simulink model "simulink_2018b"  (R2021a)
settings: Solver=ode4  StartTime=0.0  StopTime=t_f_window  FixedStep=0.0001  MaxStep=0.00002  MinStep=0.00001  RelTol=1e-7
values from neighbouring files (symbols this model uses):
  b_simulink = double(b)    [main.m]
  c_nom = double(c_nom)    [main.m]
  lambda_0_simulink = double(lambda_t_i_window)    [main.m]
  q_simulink = double(q)    [main.m]
  r_simulink = double(r)    [main.m]
  t_indices_simulink = double(t_indices_window)    [main.m]
  t_instants_simulink = double(t_window)    [main.m]
  u_nom = double(u_nom)    [main.m]
  w_pv_mean_simulink = double(w_pv_mean_window2)    [main.m]
  w_pv_real_simulink = double(w_pv(i:window+i))    [main.m]
  w_pv_simulink = double(w_pv_mean_window)    [main.m]
  w_r_mean_simulink = double(w_r_mean_window2)    [main.m]
  w_r_real_simulink = double(w_r(i:window+i))    [main.m]
  w_r_simulink = double(w_r_mean_window)    [main.m]
  w_r_variance_simulink = double(w_r_variance_window)    [main.m]
  x_t_i_simulink = double(x_t_i_window)    [main.m]
settings Model: Creator=Francesco  LastModifiedBy=emanuele
settings SolverCC: InitialStep=0.00001  AlgebraicLoopSolver=TrustRegion
settings DataIOCC: ReturnWorkspaceOutputs=off
settings DebuggingCC: SFMachineParentedDataDiag=warning  ArithmeticOperatorsInVariantConditions=warning
settings SFSimCC: CustomCodeUndefinedFunction=UseInterfaceOnly

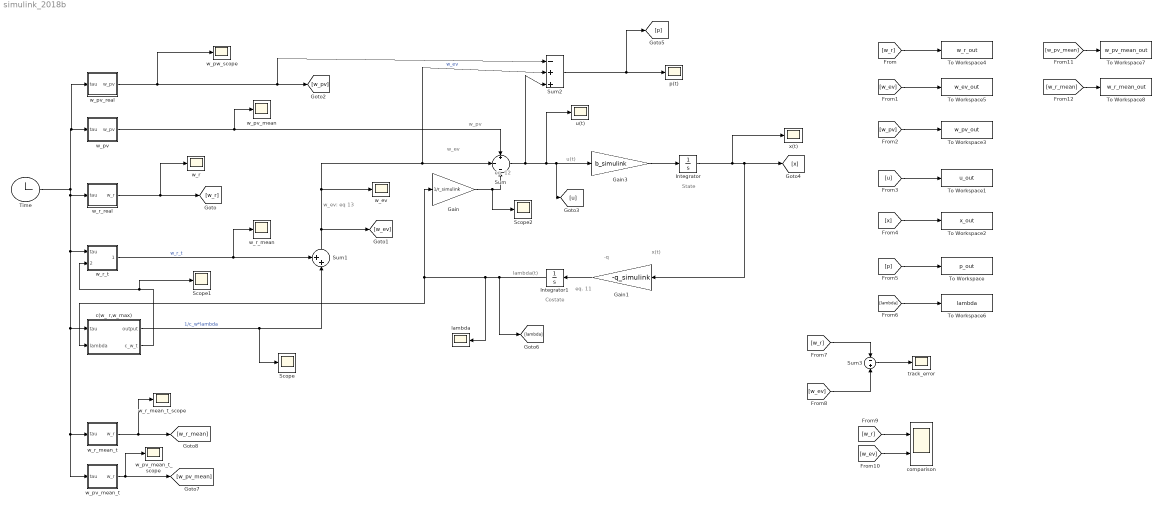
== system simulink_2018b ==
  note: w_ev:
      | eq 13
  note: eq. 11
  note: eq. 12
  note: Costate
  note: w_pv
  note: x(t)
  note: w_ev
  note: lambda(t)
  note: u(t)
  note: -q
  note: State
  Gain : Gain  Gain=1/r_simulink
  Gain1 : Gain  Gain=-q_simulink
  Gain3 : Gain  Gain=b_simulink
  Integrator : Integrator  InitialCondition=x_t_i_simulink
  Integrator1 : Integrator  InitialCondition=lambda_0_simulink
  Scope : Scope
  Scope1 : Scope
  Scope2 : Scope
  Sum : Sum  Inputs=+|-|-
  Sum1 : Sum  Inputs=++|
  Sum2 : Sum  Inputs=-++|
  Sum3 : Sum  Inputs=-+
  Time : Clock
  To Workspace : ToWorkspace  VariableName=p_out  SaveFormat=Timeseries  SampleTime=-1
  To Workspace1 : ToWorkspace  VariableName=u_out  SaveFormat=Timeseries  SampleTime=-1
  To Workspace2 : ToWorkspace  VariableName=x_out  SaveFormat=Timeseries  SampleTime=-1
  To Workspace3 : ToWorkspace  VariableName=w_pv_out  SaveFormat=Timeseries  SampleTime=-1
  To Workspace4 : ToWorkspace  VariableName=w_r_out  SaveFormat=Timeseries  SampleTime=-1
  To Workspace5 : ToWorkspace  VariableName=w_ev_out  SaveFormat=Timeseries  SampleTime=-1
  To Workspace6 : ToWorkspace  VariableName=lambda  SaveFormat=Timeseries  SampleTime=-1
  To Workspace7 : ToWorkspace  VariableName=w_pv_mean_out  SaveFormat=Timeseries  SampleTime=-1
  To Workspace8 : ToWorkspace  VariableName=w_r_mean_out  SaveFormat=Timeseries  SampleTime=-1
  c(w_ r,w_max) : MATLAB Function  TreatAsAtomicUnit=on
  comparison : Scope  NumInputPorts=2
  lambda : Scope
  p(t) : Scope
  track_error : Scope
  "u(t) " : Scope
  "w_ev " : Scope
  w_pv : MATLAB Function  TreatAsAtomicUnit=on
  w_pv_mean : Scope
  w_pv_mean_t : MATLAB Function  TreatAsAtomicUnit=on
  w_pv_mean_t_scope : Scope
  w_pv_real : MATLAB Function  TreatAsAtomicUnit=on
  w_pw_scope : Scope
  "w_r " : Scope
  w_r_mean : Scope
  w_r_mean_t : MATLAB Function  TreatAsAtomicUnit=on
  w_r_mean_t_scope : Scope
  w_r_real : MATLAB Function  TreatAsAtomicUnit=on
  w_r_t : MATLAB Function  TreatAsAtomicUnit=on
  "x(t) " : Scope
  wires:
  Gain/1 -> Scope2/1, Sum/3
  Integrator/1 -> "x(t) "/1, [x], Gain1/1
  Gain1/1 -> Integrator1/1
  Integrator1/1 -> [lambda], lambda/1, c(w_ r,w_max)/2(lambda), Gain/1
  Time/1 -> w_pv_mean_t/1(tau), w_r_mean_t/1(tau), c(w_ r,w_max)/1(tau), w_r_t/1(tau), w_r_real/1(tau), w_pv_real/1(tau), w_pv/1(tau)
  Gain3/1 -> Integrator/1
  Sum/1 -> Sum2/3, "u(t) "/1, [u], Gain3/1
  c(w_ r,w_max)/1(output) -> Scope/1, Sum1/2  "1/c_w*lambda"
  w_r_t/1(w_r_t) -> w_r_mean/1, Sum1/1  "w_r_t"
  Sum1/1 -> [w_ev], Sum2/2, Sum/2, "w_ev "/1  "w_ev"
  [w_r] -> To Workspace4/1
  [w_ev] -> To Workspace5/1
  [w_pv] -> To Workspace3/1
  [u] -> To Workspace1/1
  [x] -> To Workspace2/1
  [p] -> To Workspace/1
  Sum2/1 -> [p], p(t)/1
  w_pv/1(w_pv) -> Sum/1, w_pv_mean/1
  [lambda] -> To Workspace6/1
  Sum3/1 -> track_error/1
  [w_r] -> Sum3/1
  [w_ev] -> Sum3/2
  [w_r] -> comparison/1
  [w_ev] -> comparison/2
  c(w_ r,w_max)/2(c_w_t) -> Scope1/1, w_r_t/2(c_w_t)
  w_r_real/1(w_r) -> "w_r "/1, [w_r]
  w_pv_real/1(w_pv) -> Sum2/1, [w_pv], w_pw_scope/1
  [w_pv_mean] -> To Workspace7/1
  [w_r_mean] -> To Workspace8/1
  w_r_mean_t/1(w_r) -> w_r_mean_t_scope/1, [w_r_mean]
  w_pv_mean_t/1(w_r) -> w_pv_mean_t_scope/1, [w_pv_mean]

== matlab function simulink_2018b/w_r_t ==
  data: tau input; c_w_t input; w_r_simulink parameter; t_instants_simulink parameter; w_r_t output; t_indices_simulink parameter; c_nom parameter; u_nom parameter; w_r_variance_simulink parameter
function w_r_t = fcn(tau, c_w_t, w_r_simulink, t_instants_simulink, t_indices_simulink, c_nom, u_nom, w_r_variance_simulink)
    app=1;
    for i = 1:t_indices_simulink(end)-1
        if ( t_instants_simulink(i)<=tau )&&( tau<t_instants_simulink(i+1) )
            app = i;
            %break;
        end
    end
    E_w_r_square = w_r_simulink(app)^2 + w_r_variance_simulink(app);
    w_r_t = -(1/c_w_t)*c_nom*(E_w_r_square - (1+u_nom)*w_r_simulink(app));
    %w_r_t = w_r_simulink(app);
end

== matlab function simulink_2018b/w_pv ==
  data: tau input; w_pv output; w_pv_simulink parameter; t_instants_simulink parameter; t_indices_simulink parameter

%% profilo fotovoltaico - nullo per ora per semplicità
function w_pv = fcn(tau, w_pv_simulink, t_instants_simulink, t_indices_simulink)
    app=1;
    for i = 1:t_indices_simulink(end)-1
        if ( t_instants_simulink(i)<=tau )&&( tau<t_instants_simulink(i+1) )
            app = i;
            %break;
        end
    end
    w_pv = w_pv_simulink(app);
end

== matlab function simulink_2018b/c(w_ r,w_max) ==
  data: tau input; output output; lambda input; w_r_simulink parameter; t_indices_simulink parameter; t_instants_simulink parameter; c_w_t output; c_nom parameter; u_nom parameter
function [output, c_w_t] = fcn(tau, lambda, w_r_simulink, t_indices_simulink, t_instants_simulink, c_nom, u_nom)    
    app = 1;
    for i = 1:t_indices_simulink(end)-1
        if ( t_instants_simulink(i)<=tau )&&( tau<t_instants_simulink(i+1) )
            app = i;
        end
    end
    %c_w = assign_cw(w_r_simulink(app), p_cw_base_simulink, cw_base_simulink);
    c_w = c_nom * (1 + u_nom - w_r_simulink(app));
    output = (1/c_w)*lambda;
    c_w_t = c_w;
end
%% vedere se coeff_1 va riportato qui

== matlab function simulink_2018b/w_r_real ==
  data: tau input; w_r output; w_r_real_simulink parameter; t_instants_simulink parameter; t_indices_simulink parameter

%% profilo fotovoltaico - nullo per ora per semplicità
function w_r = fcn(tau, w_r_real_simulink, t_instants_simulink, t_indices_simulink)
    app=1;
    for i = 1:t_indices_simulink(end)-1
        if ( t_instants_simulink(i)<=tau )&&( tau<t_instants_simulink(i+1) )
            app = i;
            %break;
        end
    end
    w_r = w_r_real_simulink(app);
end

== matlab function simulink_2018b/w_pv_real ==
  data: tau input; w_pv output; w_pv_real_simulink parameter; t_instants_simulink parameter; t_indices_simulink parameter

%% profilo fotovoltaico - nullo per ora per semplicità
function w_pv = fcn(tau, w_pv_real_simulink, t_instants_simulink, t_indices_simulink)
    app=1;
    for i = 1:t_indices_simulink(end)-1
        if ( t_instants_simulink(i)<=tau )&&( tau<t_instants_simulink(i+1) )
            app = i;
            %break;
        end
    end
    w_pv = w_pv_real_simulink(app);
end

== matlab function simulink_2018b/w_r_mean_t ==
  data: tau input; w_r output; w_r_mean_simulink parameter; t_instants_simulink parameter; t_indices_simulink parameter

%% profilo fotovoltaico - nullo per ora per semplicità
function w_r = fcn(tau, w_r_mean_simulink, t_instants_simulink, t_indices_simulink)
    app=1;
    for i = 1:t_indices_simulink(end)-1
        if ( t_instants_simulink(i)<=tau )&&( tau<t_instants_simulink(i+1) )
            app = i;
            %break;
        end
    end
    w_r = w_r_mean_simulink(app);
end

== matlab function simulink_2018b/w_pv_mean_t ==
  data: tau input; w_r output; w_pv_mean_simulink parameter; t_instants_simulink parameter; t_indices_simulink parameter

%% profilo fotovoltaico - nullo per ora per semplicità
function w_r = fcn(tau, w_pv_mean_simulink, t_instants_simulink, t_indices_simulink)
    app=1;
    for i = 1:t_indices_simulink(end)-1
        if ( t_instants_simulink(i)<=tau )&&( tau<t_instants_simulink(i+1) )
            app = i;
            %break;
        end
    end
    w_r = w_pv_mean_simulink(app);
end
